simulink model "LKAS_AutoSave_DF_20220316_0937"  (R2018b)
settings: Solver=FixedStepDiscrete  StartTime=0.0  StopTime=10.0  FixedStep=0.01  RelTol=1e-3
InitFcn:
  | tmpVer = ver('MATLAB');
  | tmpVer = str2num(tmpVer.Version);
  | % -------------------------------------------------------------------
  | %  MATLAB file generated by Simulink.saveVars on 21-Nov-2019 10:06:14
  | %  MATLAB version: 7.13.0.564 (R2011b)
  | % -------------------------------------------------------------------
  | 
  | 
  | SInt16 = Simulink.AliasType;
  | SInt16.Description = 'Num';
  | if (tmpVer > 7.11)
  | 	SInt16.DataScope = 'Auto';
  | end
  | SInt16.HeaderFile = 'Rte_Type.h';
  | SInt16.BaseType = 'int16';
  | 
  | SInt32 = Simulink.AliasType;
  | SInt32.Description = 'Num';
  | if (tmpVer > 7.11)
  | 	SInt32.DataScope = 'Auto';
  | end
  | SInt32.HeaderFile = 'Rte_Type.h';
  | SInt32.BaseType = 'int32';
  | 
  | SInt8 = Simulink.AliasType;
  | SInt8.Description = 'Num';
  | if (tmpVer > 7.11)
  | 	SInt8.DataScope = 'Auto';
  | end
  | SInt8.HeaderFile = 'Rte_Type.h';
  | SInt8.BaseType = 'int8';
  | 
  | T_A_m2_1024_1_u32 = Simulink.NumericType;
  | T_A_m2_1024_1_u32.Description = 'm2 (square meters  (m2))';
  | if (tmpVer > 7.11)
  | 	T_A_m2_1024_1_u32.DataScope = 'Auto';
  | end
  | T_A_m2_1024_1_u32.HeaderFile = 'Rte_Type.h';
  | T_A_m2_1024_1_u32.DataTypeMode = 'Fixed-point: slope and bias scaling';
  | T_A_m2_1024_1_u32.SignednessBool = false;
  | T_A_m2_1024_1_u32.WordLength = 32;
  | T_A_m2_1024_1_u32.FixedExponent = -10;
  | T_A_m2_1024_1_u32.SlopeAdjustmentFactor = 1;
  | T_A_m2_1024_1_u32.Bias = 0;
  | T_A_m2_1024_1_u32.DataTypeOverride = 'Inherit';
  | T_A_m2_1024_1_u32.IsAlias = true;
  | 
  | T_A_m2_65536_1_u16 = Simulink.NumericType;
  | T_A_m2_65536_1_u16.Description = 'm2 (square meters  (m2))';
  | if (tmpVer > 7.11)
  | 	T_A_m2_65536_1_u16.DataScope = 'Auto';
  | end
  | T_A_m2_65536_1_u16.HeaderFile = 'Rte_Type.h';
  | T_A_m2_65536_1_u16.DataTypeMode = 'Fixed-point: slope and bias scaling';
  | T_A_m2_65536_1_u16.SignednessBool = false;
  | T_A_m2_65536_1_u16.WordLength = 16;
  | T_A_m2_65536_1_u16.FixedExponent = -16;
  | T_A_m2_65536_1_u16.SlopeAdjustmentFactor = 1;
  | T_A_m2_65536_1_u16.Bias = 0;
  | T_A_m2_65536_1_u16.DataTypeOverride = 'Inherit';
  | ... (+4647 lines)
StopFcn:
  | clear  T_A_m2_1024_1_u32 T_A_m2_65536_1_u16 T_A_m2_Float32 T_A_mm2_10_1_u16 T_A_mm2_4_1_s16 T_A_mm2_Float32 T_Cnt_Num_10_1_u32 T_Cnt_Num_1_1_s16 T_Cnt_Num_1_1_s32 T_Cnt_Num_1_1_s8 T_Cnt_Num_1_1_u16 T_Cnt_Num_1_1_u32 T_Cnt_Num_1_1_u8 T_E_J_1_1_s32 T_E_J_Float32 T_E_kJ_128_1_s32 T_E_kJ_Float32 T_E_kwh_10_1_u16 T_E_kwh_Float32 T_Epl_kwhpkm_100_1_u16 T_Epl_kwhpkm_Float32 T_F_N_1_1_s16 T_F_N_Float32 T_I_A_1000_1_u16 T_I_A_1048576_1_s32 T_I_A_2048_1_s16 T_I_A_32_1_s16 T_I_A_Float32 T_I_mA_1_1_s16 T_I_mA_32768_128_s16 T_I_mA_Float32 T_J_kgpm2_128_1_u16 T_J_kgpm2_Float32 T_K_NA_1000_1_s16 T_K_NA_100_1_s16 T_K_NA_100_1_u16 T_K_NA_1024_1_s16 T_K_NA_1024_1_u16 T_K_NA_128_1_s16 T_K_NA_128_1_u16 T_K_NA_128_1_u8 T_K_NA_16777216_1_u32 T_K_NA_16_1_s16 T_K_NA_16_1_u16 T_K_NA_16_1_u8 T_K_NA_1_16_u16 T_K_NA_1_1_s16 T_K_NA_1_1_u16 T_K_NA_1_1_u8 T_K_NA_32768_1_s16 T_K_NA_32768_1_u16 T_K_NA_32_1_s8 T_K_NA_4096_1_u16 T_K_NA_4194304_1_s32 T_K_NA_4194304_1_u16 T_K_NA_65536_1_s32 T_K_NA_65536_1_u16 T_K_NA_8192_1_s16 T_K_NA_8_1_s16 T_K_NA_Float32 T_M_Nm_16_1_s16 T_M_Nm_1_1_s16 T_M_Nm_32768_1_s16 T_M_Nm_32_1_s16 T_M_Nm_4_1_s16 T_M_Nm_512_1_s16 T_M_Nm_Float32 T_P_W_1_4_s16 T_P_W_1_8_s16 T_P_W_Float32 T_P_kW_128_1_s16 T_P_kW_1_8_s16 T_P_kW_8_1_s32 T_P_kW_Float32 T_Pct_pct_1024_1_s32 T_Pct_pct_1024_1_u32 T_Pct_pct_10_1_s16 T_Pct_pct_10_1_u32 T_Pct_pct_128_100_s8 T_Pct_pct_1_1_s16 T_Pct_pct_1_4_u8 T_Pct_pct_255_100_u16 T_Pct_pct_255_100_u8 T_Pct_pct_256_1_s16 T_Pct_pct_256_1_u16 T_Pct_pct_65535_100_u16 T_Pct_pct_Float32 T_R_ohm_1024_1_s16 T_R_ohm_32_1_s16 T_R_ohm_Float32 T_TK_K_16_1_s16 T_TK_K_Float32 T_T_degC_10_400_1_u16 T_T_degC_16_1_s16 T_T_degC_1_40_1_u8 T_T_degC_2_80_1_u8 T_T_degC_Float32 T_U_V_1000_1_u16 T_U_V_10_1_u8 T_U_V_200_1_u8 T_U_V_32_1_s16 T_U_V_4096_1_s16 T_U_V_512_1_s16 T_U_V_65535_8_u16 T_U_V_8192_1_u16 T_U_V_Float32 T_U_mV_1_1_s16 T_U_mV_256_20_u16 T_U_mV_Float32 T_V_l_256_1_s16 T_V_l_4096_1_s16 T_V_l_64_1_s16 T_V_l_65535_100_u16 T_V_l_Float32 T_V_ml_128_1_s16 T_V_ml_1_1_s16 T_V_ml_32768_1_s16 T_V_ml_Float32 T_V_ul_32_1_u16 T_V_ul_Float32 T_Vpl_clpkm_512_1_u16 T_Vpl_clpkm_Float32 T_a_kphps_16_1_s16 T_a_kphps_Float32 T_a_mps2_128_1_s16 T_a_mps2_Float32 T_c_MJpkg_256_1_s16 T_c_MJpkg_Float32 T_c_kJpgpK_1024_1_s16 T_c_kJpgpK_Float32 T_c_kJpkgpK_128_1_u16 T_c_kJpkgpK_Float32 T_chrg_Ah_1_1_s16 T_chrg_Ah_1_1_u16 T_chrg_Ah_1_1_u8 T_chrg_Ah_256_1_u16 T_chrg_Ah_4194304_1_s32 T_chrg_Ah_512_1_u16 T_chrg_Ah_8_1_u16 T_chrg_Ah_Float32 T_cmp_NA_100_1_s16 T_cmp_NA_128_1_s16 T_cmp_NA_16_1_s16 T_cmp_NA_32768_1_u16 T_cmp_NA_Float32 T_d2n_rpmps2_4_1_s16 T_d2n_rpmps2_Float32 T_dPct_pctps_16_1_s16 T_dPct_pctps_256_1_s16 T_dPct_pctps_Float32 T_dT_degCps_128_1_s16 T_dT_degCps_Float32 T_dV_lph_1_1_s16 T_dV_lph_Float32 T_dV_lpm_128_1_s16 T_dV_lpm_32_1_s16 T_dV_lpm_Float32 T_dV_lps_1024_1_u16 T_dV_lps_4_1_u16 T_dV_lps_Float32 T_dV_mlps_1024_1_s16 T_dV_mlps_Float32 T_d_BitField16 T_dm_gps_128_1_s16 T_dm_gps_128_1_u16 T_dm_gps_256_1_u16 T_dm_gps_Float32 T_dm_mgps_1_1_s16 T_dm_mgps_Float32 T_dn_rpmps_1_1_s16 T_dn_rpmps_2_1_s16 T_dn_rpmps_Float32 T_dp_Paps_1_1_s16 T_dp_Paps_Float32 T_dp_kPaps_1_1_s16 T_dp_kPaps_8_1_s16 T_dp_kPaps_Float32 T_dphi_degps_128_1_s16 T_dphi_degps_8_1_s16 T_dphi_degps_Float32 T_dr_ps_256_1_s16 T_dr_ps_Float32 T_drho_mgplps_1_2_s16 T_drho_mgplps_Float32 T_e_NA_1_1_u8 T_f_Hz_1_1_u16 T_f_Hz_1_1_u32 T_f_Hz_64_1_u16 T_f_Hz_8_1_s16 T_f_Hz_Float32 T_g_BitField32 T_l_km_16_1_s16 T_l_km_1_1_u16 T_l_km_1_1_u32 T_l_km_Float32 T_l_m_1024_1_s16 T_l_m_16_1_s16 T_l_m_1_1_u32 T_l_m_Float32 T_l_mm_16_1_s16 T_l_mm_1_1_u16 T_l_mm_4096_1_s16 T_l_mm_4_1_u8 T_l_mm_64_1_s16 T_l_mm_Float32 T_m_g_1_1_s16 T_m_g_2048_1_s16 T_m_g_32_1_u16 T_m_g_Float32 T_m_kg_1024_1_s16 T_m_kg_1_1_s16 T_m_kg_1_1_u32 T_m_kg_Float32 T_m_mg_128_1_s16 T_m_mg_32_1_s16 T_m_mg_Float32 T_n_rpm_1_1_s16 T_n_rpm_1_25_u8 T_n_rpm_256_50_u16 T_n_rpm_2_25_u8 T_n_rpm_4_1_u16 T_n_rpm_Float32 T_p_MPa_64_1_s16 T_p_MPa_Float32 T_p_Pa_1_1_s16 T_p_Pa_Float32 T_p_kPa_1_10_u16 T_p_kPa_1_1_s16 T_p_kPa_1_1_u8 T_p_kPa_256_1_u16 T_p_kPa_32_1_u16 T_p_kPa_64_1_s16 T_p_kPa_Float32 T_phi_deg_100_1_s16 T_phi_deg_1024_1_s16 T_phi_deg_128_1_s16 T_phi_deg_1_1_u8 T_phi_deg_256_1_s16 T_phi_deg_2_1_s8 T_phi_deg_32_1_s16 T_phi_deg_512_6_s32 T_phi_deg_Float32 T_phi_rad_2048_1_s16 T_phi_rad_Float32 T_r_NA_1024_1_s16 T_r_NA_1024_1_u16 T_r_NA_16384_1_s16 T_r_NA_16_1_s16 T_r_NA_256_1_s8 T_r_NA_256_1_u16 T_r_NA_32768_1_u16 T_r_NA_32_1_u16 T_r_NA_4096_1_s16 T_r_NA_65535_2_u16 T_r_NA_8192_1_u16 T_r_NA_Float32 T_rho_gpl_8192_1_s16 T_rho_gpl_Float32 T_rho_kgpm3_16_1_s16 T_rho_kgpm3_Float32 T_rho_mgpl_1_1_s16 T_rho_mgpl_64_1_s16 T_rho_mgpl_Float32 T_t_hour_1_1_s16 T_t_hour_Float32 T_t_m_1_1_u16 T_t_m_Float32 T_t_ms_1_1_s16 T_t_ms_1_1_u16 T_t_ms_1_1_u32 T_t_ms_4096_1_s16 T_t_ms_64_1_s16 T_t_ms_Float32 T_t_s_1000_1_s16 T_t_s_100_1_s16 T_t_s_10_1_s16 T_t_s_10_1_u16 T_t_s_1_1_s16 T_t_s_1_1_u16 T_t_s_1_1_u32 T_t_s_Float32 T_t_us_10_1_u32 T_t_us_1_1_s16 T_t_us_1_1_u32 T_t_us_1_4_u16 T_t_us_Float32 T_v_kph_1_1_u8 T_v_kph_64_1_s16 T_v_kph_64_1_u16 T_v_kph_Float32 T_v_mps_256_1_s16 T_v_mps_Float32 T_w_radps_32_1_s16 T_w_radps_Float32 T_y_BitField8 T_y_BitFieldDiagProgress T_y_BitFieldDiagStatus T_y_NA_1_1_u8 SInt16 SInt32 SInt8 T_BOOLEAN UInt16 UInt32 UInt8 s16 s32 s8 u16 u32 u8
model workspace (MAT data in the model file):
  MCOS : class17 (value not decoded)
  MCOS : class17 (value not decoded)
  MCOS : class17 (value not decoded)
  MCOS : class17 (value not decoded)
  MCOS : class17 (value not decoded)
  MCOS : class17 (value not decoded)
  MCOS : class17 (value not decoded)
  MCOS : class17 (value not decoded)
  MCOS : class17 (value not decoded)
  MCOS : class17 (value not decoded)
  MCOS : class17 (value not decoded)
  MCOS : class17 (value not decoded)
  MCOS : class17 (value not decoded)
  MCOS : class17 (value not decoded)
  MCOS : class17 (value not decoded)
  MCOS : class17 (value not decoded)
  MCOS : class17 (value not decoded)
  MCOS : class17 (value not decoded)
  MCOS : class17 (value not decoded)
  MCOS : class17 (value not decoded)
  MCOS : class17 (value not decoded)
  MCOS : class17 (value not decoded)
  MCOS : class17 (value not decoded)
  MCOS : class17 (value not decoded)
  MCOS : class17 (value not decoded)
  MCOS : class17 (value not decoded)
  MCOS : class17 (value not decoded)
  MCOS : class17 (value not decoded)
  MCOS : class17 (value not decoded)
  MCOS : class17 (value not decoded)
  MCOS : class17 (value not decoded)
  MCOS : class17 (value not decoded)
  MCOS : class17 (value not decoded)
  MCOS : class17 (value not decoded)
  MCOS : class17 (value not decoded)
  MCOS : class17 (value not decoded)
  MCOS : class17 (value not decoded)
  MCOS : class17 (value not decoded)
  MCOS : class17 (value not decoded)
  MCOS : class17 (value not decoded)
  MCOS : class17 (value not decoded)
  MCOS : class17 (value not decoded)
  MCOS : class17 (value not decoded)
  MCOS : class17 (value not decoded)
  MCOS : class17 (value not decoded)
  MCOS : class17 (value not decoded)
  MCOS : class17 (value not decoded)
  MCOS : class17 (value not decoded)
  MCOS : class17 (value not decoded)
  MCOS : class17 (value not decoded)
  MCOS : class17 (value not decoded)
  MCOS : class17 (value not decoded)
  MCOS : class17 (value not decoded)
  MCOS : class17 (value not decoded)
  MCOS : class17 (value not decoded)
  MCOS : class17 (value not decoded)
  MCOS : class17 (value not decoded)
  MCOS : class17 (value not decoded)
  MCOS : class17 (value not decoded)
  MCOS : class17 (value not decoded)
  MCOS : class17 (value not decoded)
  MCOS : class17 (value not decoded)
  MCOS : class17 (value not decoded)
  MCOS : class17 (value not decoded)
  MCOS : class17 (value not decoded)
  MCOS : class17 (value not decoded)
  MCOS : class17 (value not decoded)
  MCOS : class17 (value not decoded)
  MCOS : class17 (value not decoded)
  MCOS : class17 (value not decoded)
  MCOS : class17 (value not decoded)
  MCOS : class17 (value not decoded)
  MCOS : class17 (value not decoded)
  MCOS : class17 (value not decoded)
  MCOS : class17 (value not decoded)
  MCOS : class17 (value not decoded)
  MCOS : class17 (value not decoded)
  MCOS : class17 (value not decoded)
  MCOS : class17 (value not decoded)
  MCOS : class17 (value not decoded)
  MCOS : class17 (value not decoded)
  MCOS : class17 (value not decoded)
  MCOS : class17 (value not decoded)
  MCOS : class17 (value not decoded)
  MCOS : class17 (value not decoded)
  MCOS : class17 (value not decoded)
  MCOS : class17 (value not decoded)
  MCOS : class17 (value not decoded)
  MCOS : class17 (value not decoded)
  MCOS : class17 (value not decoded)
  MCOS : class17 (value not decoded)
  MCOS : class17 (value not decoded)
  MCOS : class17 (value not decoded)
  MCOS : class17 (value not decoded)
  MCOS : class17 (value not decoded)
  MCOS : class17 (value not decoded)
  MCOS : class17 (value not decoded)
  MCOS : class17 (value not decoded)
  MCOS : class17 (value not decoded)
  MCOS : class17 (value not decoded)
  MCOS : class17 (value not decoded)
  MCOS : class17 (value not decoded)
  MCOS : class17 (value not decoded)
  MCOS : class17 (value not decoded)
  MCOS : class17 (value not decoded)
undefined symbols (not defined in the file): LKA_CarWidth, LKA_SampleTime, LKA_StrRatio_C, LKA_Veh2CamL_C, LKA_Veh2CamW_C, LKA_WhlBaseL_C, LL_CompHdAg_C, LL_CompSWA_C, LL_CrvtPrvwT_C, LL_DesDvt_C, LL_DvtComp_C, LL_DvtPrvwT_C, LL_DvtSpdDet_vDvtSpdMin_C, LL_HandsOff_ExitTime, LL_HandsOff_TextTime, LL_HandsOff_WarnTime, LL_HdAgExT_C, LL_HdAgPrvwT_C, LL_LAccMax_C, LL_LAccRMax_C, LL_LDW_EarliestWarnLine_C, LL_LDW_LatestWarnLine_C, LL_LDWS_SUPPRESS_HEADING, LL_LFClb_TFC_FfCtlRatio_C, LL_LFClb_TFC_KdBalance_C, LL_LFClb_TFC_KdMaxSWA_C, LL_LFClb_TFC_KdV1_C, LL_LFClb_TFC_KdV2_C, LL_LFClb_TFC_KdVehSpdLwr_C, LL_LFClb_TFC_KdVehSpdUpr_C, LL_LFClb_TFC_Ki_C, LL_LFClb_TFC_KiMaxSWA_C, LL_LFClb_TFC_Kp_C, LL_LFClb_TFC_KpKlat_C, LL_LFClb_TFC_KpV1_C, LL_LFClb_TFC_KpV2_C, LL_LFClb_TFC_KpVehSpdLwr_C, LL_LFClb_TFC_KpVehSpdUpr_C, LL_LFClb_TFC_PrvwT_C, LL_LKA_EarliestWarnLine_C, LL_LKA_LatestWarnLine_C, LL_LKAExPrcs_ExitC0Dvt, LL_LKAExPrcs_ExitC0Swt, LL_LKAExPrcs_tiExitDelayTime3, LL_LKAExPrcs_tiExitTime1, LL_LKAExPrcs_tiExitTime2, LL_LKAExPrcs_tiExitTime3, LL_LKAS_OUT_OF_CONTROL_LAT_VEL, LL_LKAS_OUT_OF_CONTROL_TTLC, LL_LKASWASyn_M0, LL_LKASWASyn_M1, LL_LKASWASyn_M2, LL_LKASWASyn_M3D, LL_LKASWASyn_M3K_DT, LL_LKASWASyn_M3K_MSD, LL_LKASWASyn_SWAaddMax, LL_LKASWASyn_T2, LL_LKASWASyn_tiTrqSwaRtTime, LL_LKASWASyn_tiTrqSwaTime, LL_LKASWASyn_TrqMax ... (+46)
libraries: simulink x139, canmsglib x8, dspstat3 x3, simulink_extras x1
(part 3 of 20)

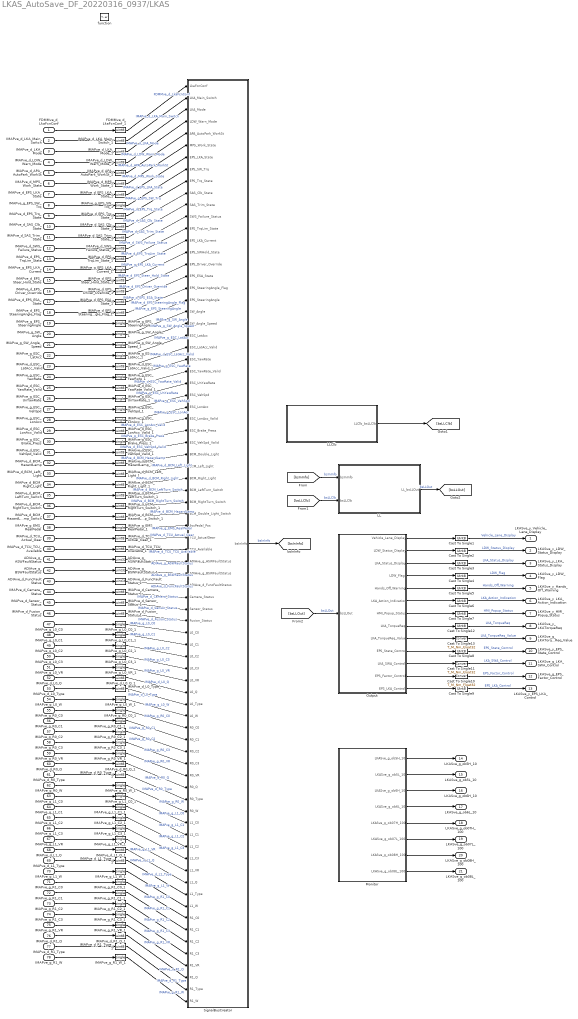
== system LKAS_AutoSave_DF_20220316_0937/LKAS ==
  FDMMve_d_LkaFcnConf : Inport
  IMAPve_d_LKA_Main_Switch : Inport  Port=2
  IMAPve_d_LKA_Mode : Inport  Port=3
  IMAPve_d_LDW_Warn_Mode : Inport  Port=4
  IMAPve_d_APA_AutoPark_WorkSt : Inport  Port=5
  IMAPve_d_MP5_Work_State : Inport  Port=6
  IMAPve_d_EPS_LKA_State : Inport  Port=7
  IMAPve_g_EPS_SW_Trq : Inport  Port=8
  IMAPve_d_EPS_Trq_State : Inport  Port=9
  IMAPve_d_SAS_Clb_State : Inport  Port=10
  IMAPve_d_SAS_Trim_State : Inport  Port=11
  IMAPve_d_SWS_Failure_Status : Inport  Port=12
  IMAPve_d_EPS_TrqLim_State : Inport  Port=13
  IMAPve_g_EPS_LKA_Current : Inport  Port=14
  IMAPve_d_EPS_Steer_Hold_State : Inport  Port=15
  IMAPve_d_EPS_Driver_Override : Inport  Port=16
  IMAPve_d_EPS_ESA_State : Inport  Port=17
  IMAPve_d_EPS_SteeringAngle_Flag : Inport  Port=18
  IMAPve_g_EPS_SteeringAngle : Inport  Port=19
  IMAPve_g_SW_Angle : Inport  Port=20
  IMAPve_g_SW_Angle_Speed : Inport  Port=21
  IMAPve_g_ESC_LatAcc : Inport  Port=22
  IMAPve_d_ESC_LatAcc_Valid : Inport  Port=23
  IMAPve_g_ESC_YawRate : Inport  Port=24
  IMAPve_d_ESC_YawRate_Valid : Inport  Port=25
  IMAPve_g_ESC_UnYawRate : Inport  Port=26
  IMAPve_g_ESC_VehSpd : Inport  Port=27
  IMAPve_g_ESC_LonAcc : Inport  Port=28
  IMAPve_d_ESC_LonAcc_Valid : Inport  Port=29
  IMAPve_g_ESC_Brake_Press : Inport  Port=30
  IMAPve_d_ESC_VehSpd_Valid : Inport  Port=31
  IMAPve_d_BCM_HazardLamp : Inport  Port=32
  IMAPve_d_BCM_Left_Light : Inport  Port=33
  IMAPve_d_BCM_Right_Light : Inport  Port=34
  IMAPve_d_BCM_LeftTurn_Switch : Inport  Port=35
  IMAPve_d_BCM_RightTurn_Switch : Inport  Port=36
  IMAPve_d_BCM_HazardLamp_Switch : Inport  Port=37
  IMAPve_g_EMS_RealPedal : Inport  Port=38
  IMAPve_d_TCU_Actual_Gear : Inport  Port=39
  IMAPve_d_TCU_TCU_Available : Inport  Port=40
  ADIAve_g_ASWFaultStatus : Inport  Port=41
  ADIAve_g_BSWFaultStatus : Inport  Port=42
  ADIAve_d_FuncFaultStatus : Inport  Port=43
  IMAPve_d_Camera_Status : Inport  Port=44
  IMAPve_d_Sensor_Status : Inport  Port=45
  IMAPve_d_Fusion_Status : Inport  Port=46
  IMAPve_g_L0_C0 : Inport  Port=47
  IMAPve_g_L0_C1 : Inport  Port=48
  IMAPve_g_L0_C2 : Inport  Port=49
  IMAPve_g_L0_C3 : Inport  Port=50
  IMAPve_g_L0_VR : Inport  Port=51
  IMAPve_d_L0_Q : Inport  Port=52
  IMAPve_d_L0_Type : Inport  Port=53
  IMAPve_g_L0_W : Inport  Port=54
  IMAPve_g_R0_C0 : Inport  Port=55
  IMAPve_g_R0_C1 : Inport  Port=56
  IMAPve_g_R0_C2 : Inport  Port=57
  IMAPve_g_R0_C3 : Inport  Port=58
  IMAPve_g_R0_VR : Inport  Port=59
  IMAPve_d_R0_Q : Inport  Port=60
  IMAPve_d_R0_Type : Inport  Port=61
  IMAPve_g_R0_W : Inport  Port=62
  IMAPve_g_L1_C0 : Inport  Port=63
  IMAPve_g_L1_C1 : Inport  Port=64
  IMAPve_g_L1_C2 : Inport  Port=65
  IMAPve_g_L1_C3 : Inport  Port=66
  IMAPve_g_L1_VR : Inport  Port=67
  IMAPve_d_L1_Q : Inport  Port=68
  IMAPve_d_L1_Type : Inport  Port=69
  IMAPve_g_L1_W : Inport  Port=70
  IMAPve_g_R1_C0 : Inport  Port=71
  IMAPve_g_R1_C1 : Inport  Port=72
  IMAPve_g_R1_C2 : Inport  Port=73
  IMAPve_g_R1_C3 : Inport  Port=74
  IMAPve_g_R1_VR : Inport  Port=75
  IMAPve_d_R1_Q : Inport  Port=76
  IMAPve_d_R1_Type : Inport  Port=77
  IMAPve_g_R1_W : Inport  Port=78
  function : TriggerPort  TriggerType=function-call  VariantControl=Variant  SampleTimeType=periodic  SampleTime=-1
  ADIAve_d_FuncFaultStatus_1 : DataTypeConversion  OutDataTypeStr=uint16
  ADIAve_g_ASWFaultStatus_1 : DataTypeConversion  OutDataTypeStr=uint32
  ADIAve_g_BSWFaultStatus_1 : DataTypeConversion  OutDataTypeStr=uint32
  Cast To Single{1..9,12} (10 alike) : DataTypeConversion  OutDataTypeStr=UInt8
  Cast To Single10 : DataTypeConversion  OutDataTypeStr=T_M_Nm_Float32
  Cast To Single11 : DataTypeConversion  OutDataTypeStr=T_M_Nm_Float32
  Cast To Single13 : DataTypeConversion  OutDataTypeStr=T_M_Nm_Float32
  FDMMve_d_LkaFcnConf_1 : DataTypeConversion  OutDataTypeStr=uint8
  IMAPve_d_APA_AutoPark_WorkSt_1 : DataTypeConversion  OutDataTypeStr=uint8
  IMAPve_d_BCM_HazardLamp_1 : DataTypeConversion  OutDataTypeStr=uint8
  IMAPve_d_BCM_HazardLamp_Switch_1 : DataTypeConversion  OutDataTypeStr=uint8
  IMAPve_d_BCM_LeftTurn_Switch_1 : DataTypeConversion  OutDataTypeStr=uint8
  IMAPve_d_BCM_Left_Light_1 : DataTypeConversion  OutDataTypeStr=uint8
  IMAPve_d_BCM_RightTurn_Switch_1 : DataTypeConversion  OutDataTypeStr=uint8
  IMAPve_d_BCM_Right_Light_1 : DataTypeConversion  OutDataTypeStr=uint8
  IMAPve_d_Camera_Status_1 : DataTypeConversion  OutDataTypeStr=uint8
  IMAPve_d_EPS_Driver_Override_1 : DataTypeConversion  OutDataTypeStr=uint8
  IMAPve_d_EPS_ESA_State_1 : DataTypeConversion  OutDataTypeStr=uint8
  IMAPve_d_EPS_LKA_State_1 : DataTypeConversion  OutDataTypeStr=uint8
  IMAPve_d_EPS_Steer_Hold_State_1 : DataTypeConversion  OutDataTypeStr=uint8
  IMAPve_d_EPS_SteeringAngle_Flag_1 : DataTypeConversion  OutDataTypeStr=uint8
  IMAPve_d_EPS_TrqLim_State_1 : DataTypeConversion  OutDataTypeStr=uint8
  IMAPve_d_EPS_Trq_State_1 : DataTypeConversion  OutDataTypeStr=uint8
  IMAPve_d_ESC_LatAcc_Valid_1 : DataTypeConversion  OutDataTypeStr=uint8
  IMAPve_d_ESC_LonAcc_Valid_1 : DataTypeConversion  OutDataTypeStr=uint8
  IMAPve_d_ESC_VehSpd_Valid_1 : DataTypeConversion  OutDataTypeStr=uint8
  IMAPve_d_ESC_YawRate_Valid_1 : DataTypeConversion  OutDataTypeStr=uint8
  IMAPve_d_Fusion_Status_1 : DataTypeConversion  OutDataTypeStr=uint8
  IMAPve_d_L0_Q_1 : DataTypeConversion  OutDataTypeStr=uint8
  IMAPve_d_L0_Type_1 : DataTypeConversion  OutDataTypeStr=uint8
  IMAPve_d_L1_Q_1 : DataTypeConversion  OutDataTypeStr=uint8
  IMAPve_d_L1_Type_1 : DataTypeConversion  OutDataTypeStr=uint8
  IMAPve_d_LDW_Warn_Mode_1 : DataTypeConversion  OutDataTypeStr=uint8
  IMAPve_d_LKA_Main_Switch_1 : DataTypeConversion  OutDataTypeStr=uint8
  IMAPve_d_LKA_Mode_1 : DataTypeConversion  OutDataTypeStr=uint8
  IMAPve_d_MP5_Work_State_1 : DataTypeConversion  OutDataTypeStr=uint8
  IMAPve_d_R0_Q_1 : DataTypeConversion  OutDataTypeStr=uint8
  IMAPve_d_R0_Type_1 : DataTypeConversion  OutDataTypeStr=uint8
  IMAPve_d_R1_Q_1 : DataTypeConversion  OutDataTypeStr=uint8
  IMAPve_d_R1_Type_1 : DataTypeConversion  OutDataTypeStr=uint8
  IMAPve_d_SAS_Clb_State_1 : DataTypeConversion  OutDataTypeStr=uint8
  IMAPve_d_SAS_Trim_State_1 : DataTypeConversion  OutDataTypeStr=uint8
  IMAPve_d_SWS_Failure_Status_1 : DataTypeConversion  OutDataTypeStr=uint8
  IMAPve_d_Sensor_Status_1 : DataTypeConversion  OutDataTypeStr=uint8
  IMAPve_d_TCU_Actual_Gear_1 : DataTypeConversion  OutDataTypeStr=uint8
  IMAPve_d_TCU_TCU_Available_1 : DataTypeConversion  OutDataTypeStr=uint8
  IMAPve_g_EMS_RealPedal_1 : DataTypeConversion  OutDataTypeStr=single
  IMAPve_g_EPS_LKA_Current_1 : DataTypeConversion  OutDataTypeStr=single
  IMAPve_g_EPS_SW_Trq_1 : DataTypeConversion  OutDataTypeStr=single
  IMAPve_g_EPS_SteeringAngle_1 : DataTypeConversion  OutDataTypeStr=single
  IMAPve_g_ESC_Brake_Press_1 : DataTypeConversion  OutDataTypeStr=single
  IMAPve_g_ESC_LatAcc_1 : DataTypeConversion  OutDataTypeStr=single
  IMAPve_g_ESC_LonAcc_1 : DataTypeConversion  OutDataTypeStr=single
  IMAPve_g_ESC_UnYawRate_1 : DataTypeConversion  OutDataTypeStr=single
  IMAPve_g_ESC_VehSpd_1 : DataTypeConversion  OutDataTypeStr=single
  IMAPve_g_ESC_YawRate_1 : DataTypeConversion  OutDataTypeStr=single
  IMAPve_g_L0_C0_1 : DataTypeConversion  OutDataTypeStr=single
  IMAPve_g_L0_C1_1 : DataTypeConversion  OutDataTypeStr=single
  IMAPve_g_L0_C2_1 : DataTypeConversion  OutDataTypeStr=single
  IMAPve_g_L0_C3_1 : DataTypeConversion  OutDataTypeStr=single
  IMAPve_g_L0_VR_1 : DataTypeConversion  OutDataTypeStr=single
  IMAPve_g_L0_W_1 : DataTypeConversion  OutDataTypeStr=single
  IMAPve_g_L1_C0_1 : DataTypeConversion  OutDataTypeStr=single
  IMAPve_g_L1_C1_1 : DataTypeConversion  OutDataTypeStr=single
  IMAPve_g_L1_C2_1 : DataTypeConversion  OutDataTypeStr=single
  IMAPve_g_L1_C3_1 : DataTypeConversion  OutDataTypeStr=single
  IMAPve_g_L1_VR_1 : DataTypeConversion  OutDataTypeStr=single
  IMAPve_g_L1_W_1 : DataTypeConversion  OutDataTypeStr=single
  IMAPve_g_R0_C0_1 : DataTypeConversion  OutDataTypeStr=single
  IMAPve_g_R0_C1_1 : DataTypeConversion  OutDataTypeStr=single
  IMAPve_g_R0_C2_1 : DataTypeConversion  OutDataTypeStr=single
  IMAPve_g_R0_C3_1 : DataTypeConversion  OutDataTypeStr=single
  IMAPve_g_R0_VR_1 : DataTypeConversion  OutDataTypeStr=single
  IMAPve_g_R0_W_1 : DataTypeConversion  OutDataTypeStr=single
  IMAPve_g_R1_C0_1 : DataTypeConversion  OutDataTypeStr=single
  IMAPve_g_R1_C1_1 : DataTypeConversion  OutDataTypeStr=single
  IMAPve_g_R1_C2_1 : DataTypeConversion  OutDataTypeStr=single
  IMAPve_g_R1_C3_1 : DataTypeConversion  OutDataTypeStr=single
  IMAPve_g_R1_VR_1 : DataTypeConversion  OutDataTypeStr=single
  IMAPve_g_R1_W_1 : DataTypeConversion  OutDataTypeStr=single
  IMAPve_g_SW_Angle_1 : DataTypeConversion  OutDataTypeStr=single
  IMAPve_g_SW_Angle_Speed_1 : DataTypeConversion  OutDataTypeStr=single
  LL : Subsystem
  LLClb : Subsystem
  Monitor : Subsystem  SystemSampleTime=0.01
  Output : Subsystem
  SignalBusCreator : Subsystem
  LKASve_y_Vehicle_Lane_Display : Outport
  LKASve_y_LDW_Status_Display : Outport  Port=2
  LKASve_y_LKA_Status_Display : Outport  Port=3
  LKASve_y_LDW_Flag : Outport  Port=4
  LKASve_y_Hands_Off_Warning : Outport  Port=5
  LKASve_y_LKA_Action_Indication : Outport  Port=6
  LKASve_y_HMI_Popup_Status : Outport  Port=7
  LKASve_y_LKATorqueReq : Outport  Port=8
  LKASve_g_LKATorqueReq_Value : Outport  Port=9
  LKASve_y_EPS_State_Control : Outport  Port=10
  LKASve_g_LKA_SWA_Control : Outport  Port=11
  LKASve_g_EPS_Factor_Control : Outport  Port=12
  LKASve_y_EPS_LKA_Control : Outport  Port=13
  LKASve_g_ob5H_10 : Outport  Port=14
  LKASve_g_ob5L_10 : Outport  Port=15
  LKASve_g_ob6H_10 : Outport  Port=16
  LKASve_g_ob6L_10 : Outport  Port=17
  LKASve_g_ob07H_100 : Outport  Port=18
  LKASve_g_ob07L_100 : Outport  Port=19
  LKASve_g_ob08H_100 : Outport  Port=20
  LKASve_g_ob08L_100 : Outport  Port=21
  wires:
  FDMMve_d_LkaFcnConf/1 -> FDMMve_d_LkaFcnConf_1/1
  FDMMve_d_LkaFcnConf_1/1 -> SignalBusCreator/1(LkaFcnConf)  "FDMMve_d_LkaFcnConf"
  IMAPve_d_LKA_Main_Switch/1 -> IMAPve_d_LKA_Main_Switch_1/1
  IMAPve_d_LKA_Main_Switch_1/1 -> SignalBusCreator/2(LKA_Main_Switch)  "IMAPve_d_LKA_Main_Switch"
  IMAPve_d_LKA_Mode/1 -> IMAPve_d_LKA_Mode_1/1
  IMAPve_d_LKA_Mode_1/1 -> SignalBusCreator/3(LKA_Mode)  "IMAPve_d_LKA_Mode"
  IMAPve_d_LDW_Warn_Mode/1 -> IMAPve_d_LDW_Warn_Mode_1/1
  IMAPve_d_LDW_Warn_Mode_1/1 -> SignalBusCreator/4(LDW_Warn_Mode)  "IMAPve_d_LDW_Warn_Mode"
  IMAPve_d_APA_AutoPark_WorkSt/1 -> IMAPve_d_APA_AutoPark_WorkSt_1/1
  IMAPve_d_APA_AutoPark_WorkSt_1/1 -> SignalBusCreator/5(APA_AutoPark_WorkSt)  "IMAPve_d_APA_AutoPark_WorkSt"
  IMAPve_d_MP5_Work_State/1 -> IMAPve_d_MP5_Work_State_1/1
  IMAPve_d_MP5_Work_State_1/1 -> SignalBusCreator/6(MP5_Work_State)  "IMAPve_d_MP5_Work_State"
  IMAPve_d_EPS_LKA_State/1 -> IMAPve_d_EPS_LKA_State_1/1
  IMAPve_d_EPS_LKA_State_1/1 -> SignalBusCreator/7(EPS_LKA_State)  "IMAPve_d_EPS_LKA_State"
  IMAPve_g_EPS_SW_Trq/1 -> IMAPve_g_EPS_SW_Trq_1/1
  IMAPve_g_EPS_SW_Trq_1/1 -> SignalBusCreator/8(EPS_SW_Trq)  "IMAPve_g_EPS_SW_Trq"
  IMAPve_d_EPS_Trq_State/1 -> IMAPve_d_EPS_Trq_State_1/1
  IMAPve_d_EPS_Trq_State_1/1 -> SignalBusCreator/9(EPS_Trq_State)  "IMAPve_d_EPS_Trq_State"
  IMAPve_d_SAS_Clb_State/1 -> IMAPve_d_SAS_Clb_State_1/1
  IMAPve_d_SAS_Clb_State_1/1 -> SignalBusCreator/10(SAS_Clb_State)  "IMAPve_d_SAS_Clb_State"
  IMAPve_d_SAS_Trim_State/1 -> IMAPve_d_SAS_Trim_State_1/1
  IMAPve_d_SAS_Trim_State_1/1 -> SignalBusCreator/11(SAS_Trim_State)  "IMAPve_d_SAS_Trim_State"
  IMAPve_d_SWS_Failure_Status/1 -> IMAPve_d_SWS_Failure_Status_1/1
  IMAPve_d_SWS_Failure_Status_1/1 -> SignalBusCreator/12(SWS_Failure_Status)  "IMAPve_d_SWS_Failure_Status"
  IMAPve_d_EPS_TrqLim_State/1 -> IMAPve_d_EPS_TrqLim_State_1/1
  IMAPve_d_EPS_TrqLim_State_1/1 -> SignalBusCreator/13(EPS_TrqLim_State)  "IMAPve_d_EPS_TrqLim_State"
  IMAPve_g_EPS_LKA_Current/1 -> IMAPve_g_EPS_LKA_Current_1/1
  IMAPve_g_EPS_LKA_Current_1/1 -> SignalBusCreator/14(EPS_LKA_Current)  "IMAPve_g_EPS_LKA_Current"
  IMAPve_d_EPS_Steer_Hold_State/1 -> IMAPve_d_EPS_Steer_Hold_State_1/1
  IMAPve_d_EPS_Steer_Hold_State_1/1 -> SignalBusCreator/15(EPS_SWHold_State)  "IMAPve_d_EPS_Steer_Hold_State"
  IMAPve_d_EPS_Driver_Override/1 -> IMAPve_d_EPS_Driver_Override_1/1
  IMAPve_d_EPS_Driver_Override_1/1 -> SignalBusCreator/16(EPS_Driver_Override)  "IMAPve_d_EPS_Driver_Override"
  IMAPve_d_EPS_ESA_State/1 -> IMAPve_d_EPS_ESA_State_1/1
  IMAPve_d_EPS_ESA_State_1/1 -> SignalBusCreator/17(EPS_ESA_State)  "IMAPve_d_EPS_ESA_State"
  IMAPve_d_EPS_SteeringAngle_Flag/1 -> IMAPve_d_EPS_SteeringAngle_Flag_1/1
  IMAPve_d_EPS_SteeringAngle_Flag_1/1 -> SignalBusCreator/18(EPS_SteeringAngle_Flag)  "IMAPve_d_EPS_SteeringAngle_Flag"
  IMAPve_g_EPS_SteeringAngle/1 -> IMAPve_g_EPS_SteeringAngle_1/1
  IMAPve_g_EPS_SteeringAngle_1/1 -> SignalBusCreator/19(EPS_SteeringAngle)  "IMAPve_g_EPS_SteeringAngle"
  IMAPve_g_SW_Angle/1 -> IMAPve_g_SW_Angle_1/1
  IMAPve_g_SW_Angle_1/1 -> SignalBusCreator/20(SW_Angle)  "IMAPve_g_SW_Angle"
  IMAPve_g_SW_Angle_Speed/1 -> IMAPve_g_SW_Angle_Speed_1/1
  IMAPve_g_SW_Angle_Speed_1/1 -> SignalBusCreator/21(SW_Angle_Speed)  "IMAPve_g_SW_Angle_Speed"
  IMAPve_g_ESC_LatAcc/1 -> IMAPve_g_ESC_LatAcc_1/1
  IMAPve_g_ESC_LatAcc_1/1 -> SignalBusCreator/22(ESC_LatAcc)  "IMAPve_g_ESC_LatAcc"
  IMAPve_d_ESC_LatAcc_Valid/1 -> IMAPve_d_ESC_LatAcc_Valid_1/1
  IMAPve_d_ESC_LatAcc_Valid_1/1 -> SignalBusCreator/23(ESC_LatAcc_Valid)  "IMAPve_d_ESC_LatAcc_Valid"
  IMAPve_g_ESC_YawRate/1 -> IMAPve_g_ESC_YawRate_1/1
  IMAPve_g_ESC_YawRate_1/1 -> SignalBusCreator/24(ESC_YawRate)  "IMAPve_g_ESC_YawRate"
  IMAPve_d_ESC_YawRate_Valid/1 -> IMAPve_d_ESC_YawRate_Valid_1/1
  IMAPve_d_ESC_YawRate_Valid_1/1 -> SignalBusCreator/25(ESC_YawRate_Valid)  "IMAPve_d_ESC_YawRate_Valid"
  IMAPve_g_ESC_UnYawRate/1 -> IMAPve_g_ESC_UnYawRate_1/1
  IMAPve_g_ESC_UnYawRate_1/1 -> SignalBusCreator/26(ESC_UnYawRate)  "IMAPve_g_ESC_UnYawRate"
  IMAPve_g_ESC_VehSpd/1 -> IMAPve_g_ESC_VehSpd_1/1
  IMAPve_g_ESC_VehSpd_1/1 -> SignalBusCreator/27(ESC_VehSpd)  "IMAPve_g_ESC_VehSpd"
  IMAPve_g_ESC_LonAcc/1 -> IMAPve_g_ESC_LonAcc_1/1
  IMAPve_g_ESC_LonAcc_1/1 -> SignalBusCreator/28(ESC_LonAcc)  "IMAPve_g_ESC_LonAcc"
  IMAPve_d_ESC_LonAcc_Valid/1 -> IMAPve_d_ESC_LonAcc_Valid_1/1
  IMAPve_d_ESC_LonAcc_Valid_1/1 -> SignalBusCreator/29(ESC_LonAcc_Valid)  "IMAPve_d_ESC_LonAcc_Valid"
  IMAPve_g_ESC_Brake_Press/1 -> IMAPve_g_ESC_Brake_Press_1/1
  IMAPve_g_ESC_Brake_Press_1/1 -> SignalBusCreator/30(ESC_Brake_Press)  "IMAPve_g_ESC_Brake_Press"
  IMAPve_d_ESC_VehSpd_Valid/1 -> IMAPve_d_ESC_VehSpd_Valid_1/1
  IMAPve_d_ESC_VehSpd_Valid_1/1 -> SignalBusCreator/31(ESC_VehSpd_Valid)  "IMAPve_d_ESC_VehSpd_Valid"
  IMAPve_d_BCM_HazardLamp/1 -> IMAPve_d_BCM_HazardLamp_1/1
  IMAPve_d_BCM_HazardLamp_1/1 -> SignalBusCreator/32(BCM_Double_Light)  "IMAPve_d_BCM_HazardLamp"
  IMAPve_d_BCM_Left_Light/1 -> IMAPve_d_BCM_Left_Light_1/1
  IMAPve_d_BCM_Left_Light_1/1 -> SignalBusCreator/33(BCM_Left_Light)  "IMAPve_d_BCM_Left_Light"
  IMAPve_d_BCM_Right_Light/1 -> IMAPve_d_BCM_Right_Light_1/1
  IMAPve_d_BCM_Right_Light_1/1 -> SignalBusCreator/34(BCM_Right_Light)  "IMAPve_d_BCM_Right_Light"
  IMAPve_d_BCM_LeftTurn_Switch/1 -> IMAPve_d_BCM_LeftTurn_Switch_1/1
  IMAPve_d_BCM_LeftTurn_Switch_1/1 -> SignalBusCreator/35(BCM_LeftTurn_Switch)  "IMAPve_d_BCM_LeftTurn_Switch"
  IMAPve_d_BCM_RightTurn_Switch/1 -> IMAPve_d_BCM_RightTurn_Switch_1/1
  IMAPve_d_BCM_RightTurn_Switch_1/1 -> SignalBusCreator/36(BCM_RightTurn_Switch)  "IMAPve_d_BCM_RightTurn_Switch"
  IMAPve_g_EMS_RealPedal/1 -> IMAPve_g_EMS_RealPedal_1/1
  IMAPve_g_EMS_RealPedal_1/1 -> SignalBusCreator/38(AccPedal_Pos)  "IMAPve_g_EMS_RealPedal"
  IMAPve_d_TCU_Actual_Gear/1 -> IMAPve_d_TCU_Actual_Gear_1/1
  IMAPve_d_TCU_Actual_Gear_1/1 -> SignalBusCreator/39(TCU_ActualGear)  "IMAPve_d_TCU_Actual_Gear"
  IMAPve_d_TCU_TCU_Available/1 -> IMAPve_d_TCU_TCU_Available_1/1
  IMAPve_d_TCU_TCU_Available_1/1 -> SignalBusCreator/40(TCU_Available)  "IMAPve_d_TCU_TCU_Available"
  IMAPve_d_Camera_Status/1 -> IMAPve_d_Camera_Status_1/1
  IMAPve_d_Camera_Status_1/1 -> SignalBusCreator/44(Camera_Status)  "IMAPve_d_Camera_Status"
  IMAPve_d_Sensor_Status/1 -> IMAPve_d_Sensor_Status_1/1
  IMAPve_d_Sensor_Status_1/1 -> SignalBusCreator/45(Sensor_Status)  "IMAPve_d_Sensor_Status"
  IMAPve_d_Fusion_Status/1 -> IMAPve_d_Fusion_Status_1/1
  IMAPve_d_Fusion_Status_1/1 -> SignalBusCreator/46(Fusion_Status)  "IMAPve_d_Fusion_Status"
  IMAPve_g_L0_C0/1 -> IMAPve_g_L0_C0_1/1
  IMAPve_g_L0_C0_1/1 -> SignalBusCreator/47(L0_C0)  "IMAPve_g_L0_C0"
  IMAPve_g_L0_C1/1 -> IMAPve_g_L0_C1_1/1
  IMAPve_g_L0_C1_1/1 -> SignalBusCreator/48(L0_C1)  "IMAPve_g_L0_C1"
  IMAPve_g_L0_C2/1 -> IMAPve_g_L0_C2_1/1
  IMAPve_g_L0_C2_1/1 -> SignalBusCreator/49(L0_C2)  "IMAPve_g_L0_C2"
  IMAPve_g_L0_C3/1 -> IMAPve_g_L0_C3_1/1
  IMAPve_g_L0_C3_1/1 -> SignalBusCreator/50(L0_C3)  "IMAPve_g_L0_C3"
  IMAPve_g_L0_VR/1 -> IMAPve_g_L0_VR_1/1
  IMAPve_g_L0_VR_1/1 -> SignalBusCreator/51(L0_VR)  "IMAPve_g_L0_VR"
  IMAPve_d_L0_Q/1 -> IMAPve_d_L0_Q_1/1
  IMAPve_d_L0_Q_1/1 -> SignalBusCreator/52(L0_Q)  "IMAPve_d_L0_Q"
  IMAPve_d_L0_Type/1 -> IMAPve_d_L0_Type_1/1
  IMAPve_d_L0_Type_1/1 -> SignalBusCreator/53(L0_Type)  "IMAPve_d_L0_Type"
  IMAPve_g_L0_W/1 -> IMAPve_g_L0_W_1/1
  IMAPve_g_L0_W_1/1 -> SignalBusCreator/54(L0_W)  "IMAPve_g_L0_W"
  IMAPve_g_R0_C0/1 -> IMAPve_g_R0_C0_1/1
  IMAPve_g_R0_C0_1/1 -> SignalBusCreator/55(R0_C0)  "IMAPve_g_R0_C0"
  IMAPve_g_R0_C1/1 -> IMAPve_g_R0_C1_1/1
  IMAPve_g_R0_C1_1/1 -> SignalBusCreator/56(R0_C1)  "IMAPve_g_R0_C1"
  IMAPve_g_R0_C2/1 -> IMAPve_g_R0_C2_1/1
  IMAPve_g_R0_C2_1/1 -> SignalBusCreator/57(R0_C2)  "IMAPve_g_R0_C2"
  IMAPve_g_R0_C3/1 -> IMAPve_g_R0_C3_1/1
  IMAPve_g_R0_C3_1/1 -> SignalBusCreator/58(R0_C3)  "IMAPve_g_R0_C3"
  IMAPve_g_R0_VR/1 -> IMAPve_g_R0_VR_1/1
  IMAPve_g_R0_VR_1/1 -> SignalBusCreator/59(R0_VR)  "IMAPve_g_R0_VR"
  IMAPve_d_R0_Q/1 -> IMAPve_d_R0_Q_1/1
  IMAPve_d_R0_Q_1/1 -> SignalBusCreator/60(R0_Q)  "IMAPve_d_R0_Q"
  IMAPve_d_R0_Type/1 -> IMAPve_d_R0_Type_1/1
  IMAPve_d_R0_Type_1/1 -> SignalBusCreator/61(R0_Type)  "IMAPve_d_R0_Type"
  IMAPve_g_R0_W/1 -> IMAPve_g_R0_W_1/1
  IMAPve_g_R0_W_1/1 -> SignalBusCreator/62(R0_W)  "IMAPve_g_R0_W"
  IMAPve_g_L1_C0/1 -> IMAPve_g_L1_C0_1/1
  IMAPve_g_L1_C0_1/1 -> SignalBusCreator/63(L1_C0)  "IMAPve_g_L1_C0"
  IMAPve_g_L1_C1/1 -> IMAPve_g_L1_C1_1/1
  IMAPve_g_L1_C1_1/1 -> SignalBusCreator/64(L1_C1)  "IMAPve_g_L1_C1"
  IMAPve_g_L1_C2/1 -> IMAPve_g_L1_C2_1/1
  IMAPve_g_L1_C2_1/1 -> SignalBusCreator/65(L1_C2)  "IMAPve_g_L1_C2"
  IMAPve_g_L1_C3/1 -> IMAPve_g_L1_C3_1/1
  IMAPve_g_L1_C3_1/1 -> SignalBusCreator/66(L1_C3)  "IMAPve_g_L1_C3"
  IMAPve_g_L1_VR/1 -> IMAPve_g_L1_VR_1/1
  IMAPve_g_L1_VR_1/1 -> SignalBusCreator/67(L1_VR)  "IMAPve_g_L1_VR"
  IMAPve_d_L1_Q/1 -> IMAPve_d_L1_Q_1/1
  IMAPve_d_L1_Q_1/1 -> SignalBusCreator/68(L1_Q)  "IMAPve_d_L1_Q"
  IMAPve_d_L1_Type/1 -> IMAPve_d_L1_Type_1/1
  IMAPve_d_L1_Type_1/1 -> SignalBusCreator/69(L1_Type)  "IMAPve_d_L1_Type"
  IMAPve_g_L1_W/1 -> IMAPve_g_L1_W_1/1
  IMAPve_g_L1_W_1/1 -> SignalBusCreator/70(L1_W)  "IMAPve_g_L1_W"
  IMAPve_g_R1_C0/1 -> IMAPve_g_R1_C0_1/1
  IMAPve_g_R1_C0_1/1 -> SignalBusCreator/71(R1_C0)  "IMAPve_g_R1_C0"
  IMAPve_g_R1_C1/1 -> IMAPve_g_R1_C1_1/1
  IMAPve_g_R1_C1_1/1 -> SignalBusCreator/72(R1_C1)  "IMAPve_g_R1_C1"
  IMAPve_g_R1_C2/1 -> IMAPve_g_R1_C2_1/1
  IMAPve_g_R1_C2_1/1 -> SignalBusCreator/73(R1_C2)  "IMAPve_g_R1_C2"
  IMAPve_g_R1_C3/1 -> IMAPve_g_R1_C3_1/1
  IMAPve_g_R1_C3_1/1 -> SignalBusCreator/74(R1_C3)  "IMAPve_g_R1_C3"
  IMAPve_g_R1_VR/1 -> IMAPve_g_R1_VR_1/1
  IMAPve_g_R1_VR_1/1 -> SignalBusCreator/75(R1_VR)  "IMAPve_g_R1_VR"
  IMAPve_d_R1_Q/1 -> IMAPve_d_R1_Q_1/1
  IMAPve_d_R1_Q_1/1 -> SignalBusCreator/76(R1_Q)  "IMAPve_d_R1_Q"
  IMAPve_d_R1_Type/1 -> IMAPve_d_R1_Type_1/1
  IMAPve_d_R1_Type_1/1 -> SignalBusCreator/77(R1_Type)  "IMAPve_d_R1_Type"
  IMAPve_g_R1_W/1 -> IMAPve_g_R1_W_1/1
  IMAPve_g_R1_W_1/1 -> SignalBusCreator/78(R1_W)  "IMAPve_g_R1_W"
  Monitor/1(LKASve_g_ob5H_10) -> LKASve_g_ob5H_10/1
  Monitor/8(LKASve_g_ob08L_100) -> LKASve_g_ob08L_100/1
  Monitor/7(LKASve_g_ob08H_100) -> LKASve_g_ob08H_100/1
  [bsLLOut] -> Output/1(bsLLOut)  "bsLLOut"
  Monitor/6(LKASve_g_ob07L_100) -> LKASve_g_ob07L_100/1
  Monitor/3(LKASve_g_ob6H_10) -> LKASve_g_ob6H_10/1
  [bsLLClb] -> LL/2(bsLLClb)  "bsLLClb"
  LL/1(LL_bsLLOut) -> [bsLLOut]  "bsLLOut"
  LLClb/1(LLClb_bsLLClb) -> [bsLLClb]
  SignalBusCreator/1(bsInInfo) -> [bsInInfo]  "bsInInfo"
  Monitor/4(LKASve_g_ob6L_10) -> LKASve_g_ob6L_10/1
  Monitor/5(LKASve_g_ob07H_100) -> LKASve_g_ob07H_100/1
  [bsInInfo] -> LL/1(bsInInfo)  "bsInInfo"
  Monitor/2(LKASve_g_ob5L_10) -> LKASve_g_ob5L_10/1
  Output/1(Vehicle_Lane_Display) -> Cast To Single1/1
  Output/2(LDW_Status_Display) -> Cast To Single2/1
  Output/3(LKA_Status_Display) -> Cast To Single3/1
  Output/4(LDW_Flag) -> Cast To Single4/1
  Output/5(Hands_Off_Warning) -> Cast To Single5/1
  Output/6(LKA_Action_Indication) -> Cast To Single6/1
  Output/7(HMI_Popup_Status) -> Cast To Single7/1
  Output/8(LKA_TorqueReq) -> Cast To Single12/1
  Output/9(LKA_TorqueReq_Value) -> Cast To Single13/1
  Output/10(EPS_State_Control) -> Cast To Single8/1
  Output/11(LKA_SWA_Control) -> Cast To Single11/1
  Output/12(EPS_Factor_Control) -> Cast To Single10/1
  Output/13(EPS_LKA_Control) -> Cast To Single9/1
  Cast To Single1/1 -> LKASve_y_Vehicle_Lane_Display/1  "Vehicle_Lane_Display"
  Cast To Single2/1 -> LKASve_y_LDW_Status_Display/1  "LDW_Status_Display"
  Cast To Single3/1 -> LKASve_y_LKA_Status_Display/1  "LKA_Status_Display"
  Cast To Single4/1 -> LKASve_y_LDW_Flag/1  "LDW_Flag"
  Cast To Single5/1 -> LKASve_y_Hands_Off_Warning/1  "Hands_Off_Warning"
  Cast To Single6/1 -> LKASve_y_LKA_Action_Indication/1  "LKA_Action_Indication"
  Cast To Single7/1 -> LKASve_y_HMI_Popup_Status/1  "HMI_Popup_Status"
  Cast To Single12/1 -> LKASve_y_LKATorqueReq/1  "LKA_TorqueReq"
  Cast To Single13/1 -> LKASve_g_LKATorqueReq_Value/1  "LKA_TorqueReq_Value"
  Cast To Single8/1 -> LKASve_y_EPS_State_Control/1  "EPS_State_Control"
  Cast To Single11/1 -> LKASve_g_LKA_SWA_Control/1  "LKA_SWA_Control"
  Cast To Single10/1 -> LKASve_g_EPS_Factor_Control/1  "EPS_Factor_Control"
  Cast To Single9/1 -> LKASve_y_EPS_LKA_Control/1  "EPS_LKA_Control"
  ADIAve_g_ASWFaultStatus/1 -> ADIAve_g_ASWFaultStatus_1/1
  ADIAve_g_BSWFaultStatus/1 -> ADIAve_g_BSWFaultStatus_1/1
  ADIAve_d_FuncFaultStatus/1 -> ADIAve_d_FuncFaultStatus_1/1
  ADIAve_g_ASWFaultStatus_1/1 -> SignalBusCreator/41(ADIAve_g_ASWFaultStatus)  "ADIAve_g_ASWFaultStatus"
  ADIAve_g_BSWFaultStatus_1/1 -> SignalBusCreator/42(ADIAve_g_BSWFaultStatus)  "ADIAve_g_BSWFaultStatus"
  ADIAve_d_FuncFaultStatus_1/1 -> SignalBusCreator/43(ADIAve_d_FuncFaultStatus)  "ADIAve_d_FuncFaultStatus"
  IMAPve_d_BCM_HazardLamp_Switch_1/1 -> SignalBusCreator/37(BCM_Double_Light_Switch)  "IMAPve_d_BCM_HazardLamp"
  IMAPve_d_BCM_HazardLamp_Switch/1 -> IMAPve_d_BCM_HazardLamp_Switch_1/1

== system LKAS_AutoSave_DF_20220316_0937/LKAS/LL ==
  bsInInfo : Inport
  bsLLClb : Inport  Port=2
  Bus Selector : BusSelector  OutputSignals=bsMP5Info.LKA_Mode
  Bus Selector1 : BusSelector  OutputSignals=bsLaneInfo.bsR0Info.R0_Q,bsLaneInfo.bsL0Info.L0_Q
  Bus Selector2 : BusSelector  OutputSignals=bsEPSInfo
  Bus Selector3 : BusSelector  OutputSignals=LKA_State,LDW_State
  Bus Selector4 : BusSelector  OutputSignals=bsLaneInfo.Fusion_AdditionalInf.Carema_Status
  Bus Selector5 : BusSelector  OutputSignals=bsMP5Info.LKA_Mode
  Fault_Diagnostic : Subsystem
  Ground1 : Ground
  Human Machine Interface (HMI) : Subsystem
  LL Inputs Mapping : Subsystem
  LLOn : Subsystem
  LLOut : Subsystem
  Terminator : Terminator
  Version : Constant  Value=220316  OutMin=20410  OutMax=220630  OutDataTypeStr=single
  LL_bsLLOut : Outport
      settings: AttributesFormatString=Disable Action: %<OutputWhenDisabled>
  tag scope: LLMon=global
  wires:
  [LLOn_bsLDWWarnInfo] -> Human Machine Interface (HMI)/4(HMI_LDWWarn)
  Bus Selector2/1 -> Human Machine Interface (HMI)/7(HMI_EPSInfo)  "<bsEPSInfo>"
  Bus Selector1/2 -> Human Machine Interface (HMI)/6(HMI_L0_Quality)  "<L0_Q>"
  Bus Selector1/1 -> Human Machine Interface (HMI)/5(HMI_R0_Quality)  "<R0_Q>"
  Bus Selector5/1 -> Human Machine Interface (HMI)/1(HMI_stDACmode)  "<LKA_Mode>"
  [LLOn_bsLLState] -> Bus Selector3/1
  Bus Selector4/1 -> Human Machine Interface (HMI)/9(HMI_Front_Camera_Blocked)  "<Carema_Status>"
  Ground1/1 -> Human Machine Interface (HMI)/8(HMI_camera_common_fault)
  Bus Selector3/1 -> Human Machine Interface (HMI)/2(HMI_LKA_STATE)  "<LKA_State>"
  Bus Selector3/2 -> Human Machine Interface (HMI)/3(HMI_LDW_STATE)  "<LDW_State>"
  [bsInfo] -> Bus Selector5/1, Bus Selector1/1, Bus Selector2/1, Bus Selector4/1
  [LLOn_phiSWACmd] -> LLOut/2(LLOut_phiSWACmd)
  [bsInfo] -> LLOut/5(LLOut_bsInfo)
  [LLOn_M] -> LLOut/4(LLOut_M)
  [LLOn_bsLLState] -> LLOut/1(LLOut_bsLLState)
  LLOut/1(LL_bsLLOut) -> LL_bsLLOut/1
  [HMI_bsLLHMI] -> LLOut/3(LLOut_bsLLHMI)
  Bus Selector/1 -> LLOn/Enable  "<LKA_Mode>"
  bsInInfo/1 -> [bsInInfo]
  Human Machine Interface (HMI)/1(HMI_LDWLKA) -> [HMI_bsLLHMI]  "bsLLHMI"
  Version/1 -> Terminator/1  "ob_LKA_Version"
  LLOn/2(LDW_Flag) -> [LLOn_bsLDWWarnInfo]
  bsLLClb/1 -> [bsLLClb]
  LLOn/1(bsLLState) -> [LLOn_bsLLState]
  LLOn/3(phiSWACmd) -> [LLOn_phiSWACmd]
  LLOn/4(M) -> [LLOn_M]
  LLOn/5(LLMon) -> [LLMon]
  Fault_Diagnostic/1(bsSignalFault) -> [bsSignalFault]
  [bsInInfo] -> Fault_Diagnostic/1(bsInInfo)
  LL Inputs Mapping/1(bsInfo) -> [bsInfo]
  [bsInInfo] -> LL Inputs Mapping/1(bsInInfo)
  [bsInfo] -> Bus Selector/1, LLOn/1(bsInInfo)
  [bsLLClb] -> LLOn/2(bsLLClb)
  [bsSignalFault] -> LLOn/3(bsSignalFault)
  [bsLLClb] -> Human Machine Interface (HMI)/10(HMI_bsLLClb)
  [bsLLClb] -> LL Inputs Mapping/2(bsLLClb)

== system LKAS_AutoSave_DF_20220316_0937/LKAS/LLClb ==
  Bus Creator : BusCreator  Inputs=4
  ConstantClb : Subsystem
  LDWClb : Subsystem
  LKAClb : Subsystem
  LLSMConClb : Subsystem
  LLClb_bsLLClb : Outport
  wires:
  ConstantClb/1(ConstantClb) -> Bus Creator/4  "bsConstantClb"
  LLSMConClb/1(LLSMConClb) -> Bus Creator/1  "bsLLSMConClb"
  Bus Creator/1 -> LLClb_bsLLClb/1  "bsLLClb"
  LDWClb/1(LDWClb) -> Bus Creator/2  "bsLDWClb"
  LKAClb/1(LKAClb) -> Bus Creator/3  "bsLKAClb"
